simulink model "exampleBasicCreateTHB"  (R2013b)
settings: Solver=VariableStepDiscrete  StartTime=0.0  StopTime=10.0  MaxStep=0.1  RelTol=1e-3
libraries: simulink x2, carnot x1
settings Model: Creator=drhf  LastModifiedBy=drhf
settings OptimizationCC: InlineParams=on

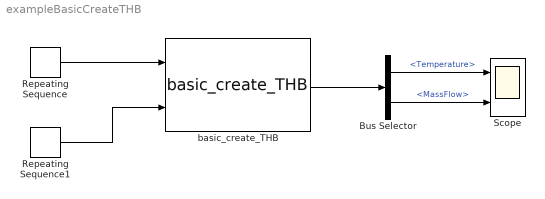
== system exampleBasicCreateTHB ==
  Bus Selector : BusSelector  OutputSignals=Temperature,MassFlow
  Repeating Sequence : simulink/Sources/Repeating Sequence  rep_seq_t=[0 5 10]  rep_seq_y=[0 600 0]/3600
  Repeating Sequence1 : simulink/Sources/Repeating Sequence  rep_seq_t=[0 5 10]  rep_seq_y=[20 40 20]
  Scope : Scope  NumInputPorts=2
      settings: YMin=-5~-5  YMax=5~5
  basic_create_THB : carnot/Basic/Hydraulics/basic_create_THB  p=2e5  fluid=1  mix=0  dia=0.03  hgt=0  mID=1
  wires:
  Repeating Sequence/1 -> basic_create_THB/1
  Repeating Sequence1/1 -> basic_create_THB/2
  basic_create_THB/1 -> Bus Selector/1
  Bus Selector/1 -> Scope/1  "<Temperature>"
  Bus Selector/2 -> Scope/2  "<MassFlow>"
